simulink model "wqRL_multi_bal_system"  (R2021a)
settings: Solver=ode23t  StartTime=0.0  StopTime=Inf  FixedStep=0.02  RelTol=1e-3  AbsTol=1e-3
undefined symbols (not defined in the file or in its folder): dphi0, dtheta0, phi0, Tf, theta0, Ts
libraries: angle_lib x4, simulink_extras x2, pendulumLib x1, rllib x1, simulink x1
settings Model: DataDictionary=rl_data.sldd  Creator=tshintai  LastModifiedBy=WQ
settings SolverCC: AutoScaleAbsTol=off
settings ExplorerConfigSet: InternalSimMechanicsExplorerSettings="<ExplorerConfiguration><canonicalview>default</canonicalview><AnimationSetting><BasePlaybackSpeed>1.0</BasePlaybackSpeed><PlaybackSpeedFactor>1.0</PlaybackSpeedFactor></AnimationSetting><TilePanel><TileInfo><Tiles Columns=\"1\" Count=\"1\" Rows=\"1\"><Column Weight=\"1\"/><Row Weight=\"1\"/><Tile Height=\"1\" Width=\"1\" X=\"0\" Y=\"0\"/></Tiles></TileInfo><SceneInfo><SceneViewer><BGColor><R>0.60000002384185791</R><G>0.60000002384185791</G><B>0.60000002384185791</B></BGColor><Camera><DoPerspective>on</DoPerspective><Position><X>0.334156231583514596</X><Y>0.107146061295956732</Y><Z>0.154419804164132285</Z></Position><Center><X>0.145480827141795971</X><Y>0.0537418892551446009</Y><Z>0.077934111254939889</Z></Center><Up><X>-0.332530024195597795</X><Y>-0.157027945704575345</Y><Z>0.929927958110882913</Z></Up><ViewLimDist>1</ViewLimDist><YLim>0.466307658154998583</YLim><XLim>0.535390274177961367</XLim></Camera></SceneViewer></SceneInfo></TilePanel><MechEditorPanel><Cameras><Camera><Id>Camera1</Id><Value><Name>Camera1</Name><NativeCamera><PositionKeyframeSet/><CenterKeyframeSet/><UpVectorKeyframeSet/></NativeCamera></Value></Camera></Cameras><GfxPanelCameraMap><MapElement CameraMLId=\"Camera1\" GfxPanelIndex=\"0\"/></GfxPanelCameraMap><VideoCreator><PlaybackSpeedRatio>1.0</PlaybackSpeedRatio><FrameRate>30</FrameRate><VideoFormat>Motion JPEG AVI</VideoFormat><FrameSize>auto</FrameSize></VideoCreator></MechEditorPanel></ExplorerConfiguration>"

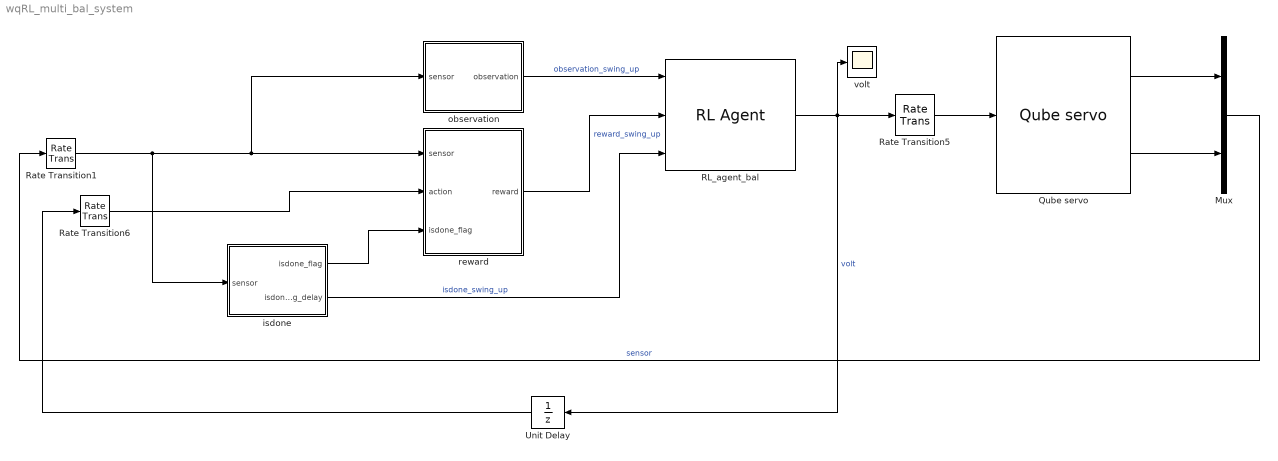
== system wqRL_multi_bal_system ==
  Mux : Mux  Inputs=2
  Qube servo : pendulumLib/Qube servo  a0=[theta0, phi0]  w0=[dtheta0, dphi0]  R_m=R_m  L_m=L_m  mu_m=mu_m  K_b=K_b_2  n=n  rod_mass=m_r  rod_length=L_r  rod_rad=rod_rad  p_mass=m_p  p_length=L_p  p_rad=p_rad  D_r=D_r_2  D_p=D_p
  RL_agent_bal : rllib/RL Agent  Agent=agent_bal  ExternalActionAsInput=off  ProvideCumRwd=off  TreatAsDirectFeedthrough=on
  Rate Transition1 : RateTransition  OutPortSampleTime=Ts
  Rate Transition5 : RateTransition
  Rate Transition6 : RateTransition  OutPortSampleTime=Ts
  Unit Delay : UnitDelay  SampleTime=-1  HasFrameUpgradeWarning=on
  isdone : Subsystem  VariantControl=VARIANT_INV_POS
  "observation " : Subsystem  VariantControl=VARIANT_OBS_ARM_PEND
  reward : Subsystem  VariantControl=VARIANT_INV_POS
  volt : Scope
  wires:
  Qube servo/1 -> Mux/1
  Qube servo/2 -> Mux/2
  Mux/1 -> Rate Transition1/1  "sensor"
  RL_agent_bal/1 -> Unit Delay/1, volt/1, Rate Transition5/1  "volt"
  Rate Transition5/1 -> Qube servo/1
  Unit Delay/1 -> Rate Transition6/1
  "observation "/1(observation) -> RL_agent_bal/1  "observation_swing_up"
  reward/1(reward) -> RL_agent_bal/2  "reward_swing_up"
  Rate Transition6/1 -> reward/2(action)
  isdone/2(isdone_flag_delay) -> RL_agent_bal/3  "isdone_swing_up"
  Rate Transition1/1 -> reward/1(sensor), "observation "/1(sensor), isdone/1(sensor)
  isdone/1(isdone_flag) -> reward/3(isdone_flag)

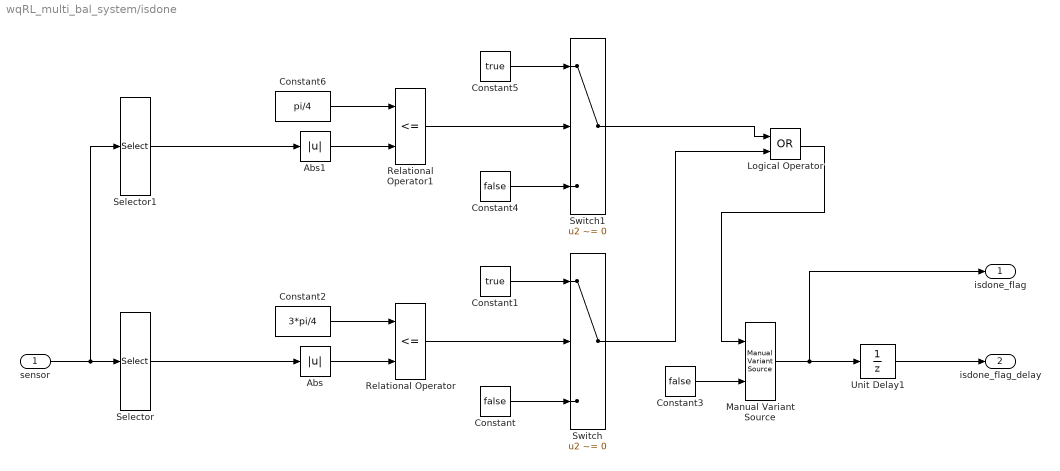
== system wqRL_multi_bal_system/isdone ==
  sensor : Inport
  Abs : Abs
  Abs1 : Abs
  Constant : Constant  Value=false
  Constant1 : Constant  Value=true
  Constant2 : Constant  Value=3*pi/4
  Constant3 : Constant  Value=false
  Constant4 : Constant  Value=false
  Constant5 : Constant  Value=true
  Constant6 : Constant  Value=pi/4
  Logical Operator : Logic  Operator=OR  AllPortsSameDT=off  OutDataTypeStr=boolean
  Manual Variant Source : simulink/Signal Routing/Manual Variant Source  NumChoices=2  LabelModeActiveChoice=V_2
  Relational Operator : RelationalOperator  Operator=<=  OutDataTypeStr=boolean  RndMeth=Simplest
  Relational Operator1 : RelationalOperator  Operator=<=  OutDataTypeStr=boolean  RndMeth=Simplest
  Selector : Selector  InputPortWidth=4  IndexOptions=Index vector (dialog)  Indices=[1]  OutputSizes=1
  Selector1 : Selector  InputPortWidth=4  IndexOptions=Index vector (dialog)  Indices=[2]  OutputSizes=1
  Switch : Switch  Criteria=u2 ~= 0
  Switch1 : Switch  Criteria=u2 ~= 0
  Unit Delay1 : UnitDelay  SampleTime=-1  HasFrameUpgradeWarning=on
  isdone_flag : Outport
  isdone_flag_delay : Outport  Port=2
  wires:
  Constant2/1 -> Relational Operator/1
  Constant/1 -> Switch/3
  Relational Operator/1 -> Switch/2
  Abs/1 -> Relational Operator/2
  Constant1/1 -> Switch/1
  Selector/1 -> Abs/1
  Switch/1 -> Logical Operator/2
  Manual Variant Source/1 -> isdone_flag/1, Unit Delay1/1
  Constant3/1 -> Manual Variant Source/2
  Unit Delay1/1 -> isdone_flag_delay/1
  Constant5/1 -> Switch1/1
  Switch1/1 -> Logical Operator/1
  Abs1/1 -> Relational Operator1/2
  Constant6/1 -> Relational Operator1/1
  Constant4/1 -> Switch1/3
  Relational Operator1/1 -> Switch1/2
  Selector1/1 -> Abs1/1
  sensor/1 -> Selector1/1, Selector/1
  Logical Operator/1 -> Manual Variant Source/1

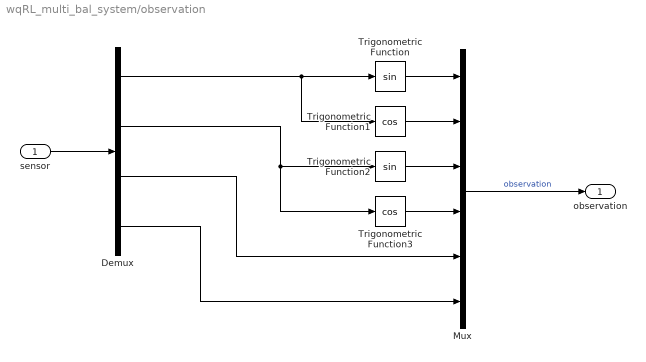
== system wqRL_multi_bal_system/observation  ==
  sensor : Inport
  Demux : Demux
  Mux : Mux  Inputs=6
  Trigonometric Function : Trigonometry
  Trigonometric Function1 : Trigonometry  Operator=cos
  Trigonometric Function2 : Trigonometry
  Trigonometric Function3 : Trigonometry  Operator=cos
  observation : Outport
  wires:
  Demux/4 -> Mux/6
  Demux/2 -> Trigonometric Function2/1, Trigonometric Function3/1
  Trigonometric Function3/1 -> Mux/4
  Trigonometric Function2/1 -> Mux/3
  sensor/1 -> Demux/1
  Mux/1 -> observation/1  "observation"
  Trigonometric Function/1 -> Mux/1
  Trigonometric Function1/1 -> Mux/2
  Demux/1 -> Trigonometric Function/1, Trigonometric Function1/1
  Demux/3 -> Mux/5

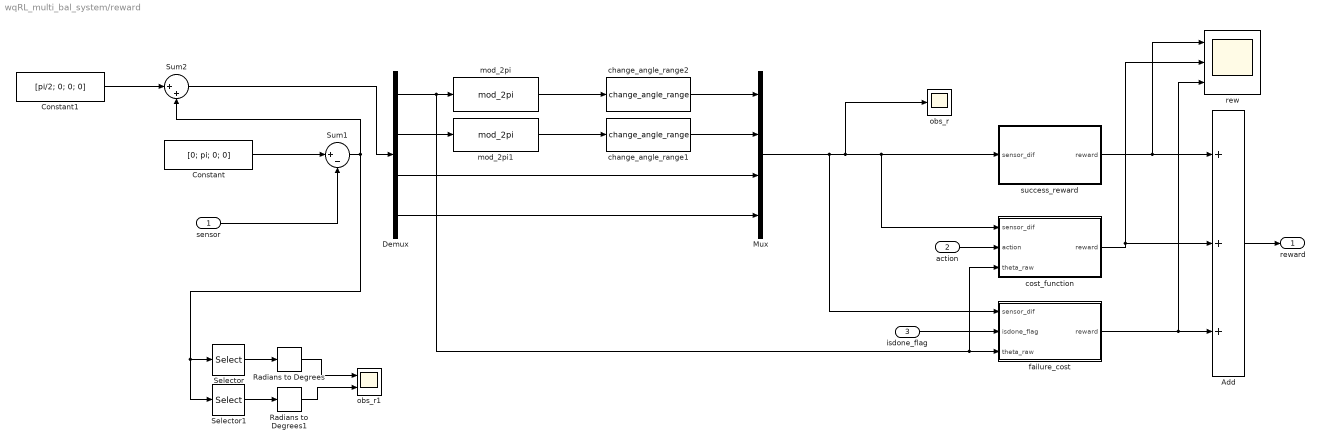
== system wqRL_multi_bal_system/reward ==
  sensor : Inport
  action : Inport  Port=2
  isdone_flag : Inport  Port=3
  Add : Sum  Inputs=+++
  Constant : Constant  Value=[0; pi; 0; 0]
  Constant1 : Constant  Value=[pi/2; 0; 0; 0]
  Demux : Demux
  Mux : Mux
  Radians to Degrees : simulink_extras/Transformations/Radians to Degrees
  Radians to Degrees1 : simulink_extras/Transformations/Radians to Degrees
  Selector : Selector  InputPortWidth=4  IndexOptions=Index vector (dialog)  Indices=[1]  OutputSizes=1
  Selector1 : Selector  InputPortWidth=4  IndexOptions=Index vector (dialog)  Indices=[2]  OutputSizes=1
  Sum1 : Sum  Inputs=|+-
  Sum2 : Sum  Inputs=|++
  change_angle_range1 : angle_lib/change_angle_range  SystemSampleTime=-1  VariantActivationTime=update diagram  Latency=0  AutoFrameSizeCalculation=off
  change_angle_range2 : angle_lib/change_angle_range  SystemSampleTime=-1  VariantActivationTime=update diagram  Latency=0  AutoFrameSizeCalculation=off
  cost_function : Subsystem
  failure_cost : Subsystem
  mod_2pi : angle_lib/mod_2pi  SystemSampleTime=-1  VariantActivationTime=update diagram  Latency=0  AutoFrameSizeCalculation=off
  mod_2pi1 : angle_lib/mod_2pi  SystemSampleTime=-1  VariantActivationTime=update diagram  Latency=0  AutoFrameSizeCalculation=off
  obs_r : Scope
  obs_r1 : Scope  NumInputPorts=2
  rew : Scope  NumInputPorts=3
  success_reward : Subsystem
  reward : Outport
  wires:
  isdone_flag/1 -> failure_cost/2(isdone_flag)
  failure_cost/1(reward) -> rew/3, Add/3
  success_reward/1(reward) -> rew/1, Add/1
  cost_function/1(reward) -> rew/2, Add/2
  action/1 -> cost_function/2(action)
  Add/1 -> reward/1
  Mux/1 -> cost_function/1(sensor_dif), success_reward/1(sensor_dif), obs_r/1, failure_cost/1(sensor_dif)
  Demux/2 -> mod_2pi1/1
  change_angle_range2/1 -> Mux/1
  change_angle_range1/1 -> Mux/2
  Demux/3 -> Mux/3
  Demux/4 -> Mux/4
  mod_2pi/1 -> change_angle_range2/1
  mod_2pi1/1 -> change_angle_range1/1
  Demux/1 -> failure_cost/3(theta_raw), cost_function/3(theta_raw), mod_2pi/1
  Radians to Degrees/1 -> obs_r1/1
  Radians to Degrees1/1 -> obs_r1/2
  Selector1/1 -> Radians to Degrees1/1
  Selector/1 -> Radians to Degrees/1
  sensor/1 -> Sum1/2
  Constant/1 -> Sum1/1
  Constant1/1 -> Sum2/1
  Sum1/1 -> Sum2/2, Selector1/1, Selector/1
  Sum2/1 -> Demux/1

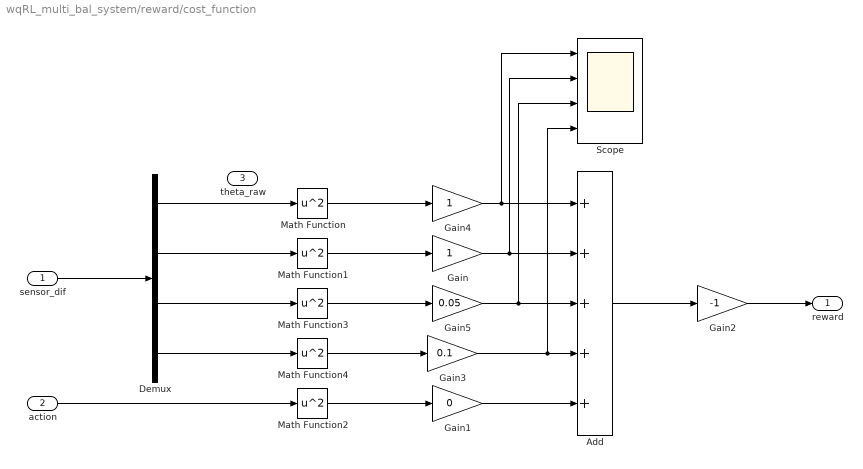
== system wqRL_multi_bal_system/reward/cost_function ==
  sensor_dif : Inport
  action : Inport  Port=2
  theta_raw : Inport  Port=3
  Add : Sum  Inputs=+++++
  Demux : Demux
  Gain : Gain
  Gain1 : Gain  Gain=0
  Gain2 : Gain  Gain=-1
  Gain3 : Gain  Gain=0.1
  Gain4 : Gain
  Gain5 : Gain  Gain=0.05
  Math Function{,1..4} (5 alike) : Math  Operator=square  SaturateOnIntegerOverflow=on
  Scope : Scope  NumInputPorts=4
  reward : Outport
  wires:
  Math Function4/1 -> Gain3/1
  Gain4/1 -> Scope/1, Add/1
  Gain/1 -> Scope/2, Add/2
  Gain5/1 -> Scope/3, Add/3
  Gain3/1 -> Scope/4, Add/4
  Gain1/1 -> Add/5
  Gain2/1 -> reward/1
  Add/1 -> Gain2/1
  sensor_dif/1 -> Demux/1
  Demux/4 -> Math Function4/1
  Demux/3 -> Math Function3/1
  Demux/2 -> Math Function1/1
  Math Function1/1 -> Gain/1
  Math Function3/1 -> Gain5/1
  action/1 -> Math Function2/1
  Demux/1 -> Math Function/1
  Math Function/1 -> Gain4/1
  Math Function2/1 -> Gain1/1

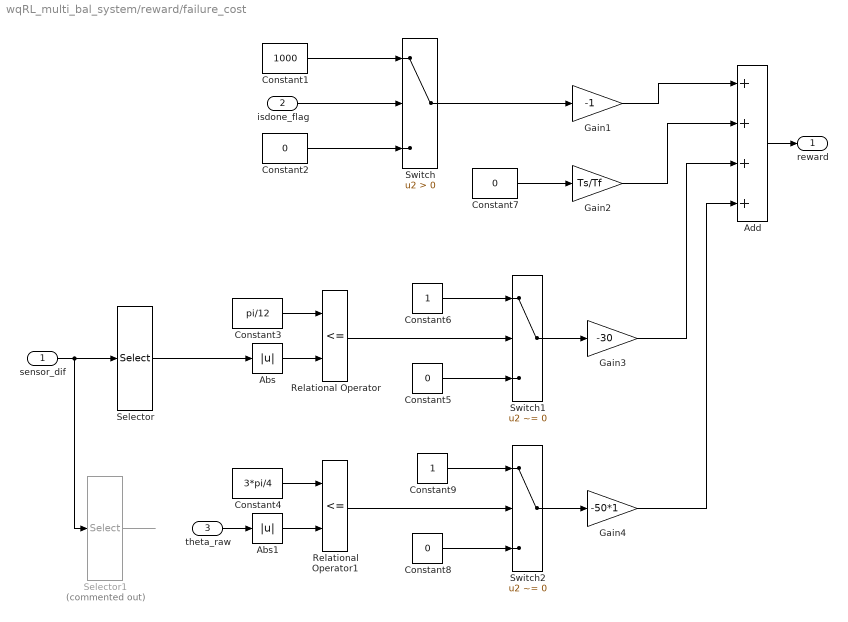
== system wqRL_multi_bal_system/reward/failure_cost ==
  sensor_dif : Inport
  isdone_flag : Inport  Port=2
  theta_raw : Inport  Port=3
  Abs : Abs
  Abs1 : Abs
  Add : Sum  Inputs=++++
  Constant1 : Constant  Value=1000
  Constant{2,5,7..8} (4 alike) : Constant  Value=0
  Constant3 : Constant  Value=pi/12
  Constant4 : Constant  Value=3*pi/4
  Constant6 : Constant
  Constant9 : Constant
  Gain1 : Gain  Gain=-1
  Gain2 : Gain  Gain=Ts/Tf
  Gain3 : Gain  Gain=-30
  Gain4 : Gain  Gain=-50*1
  Relational Operator : RelationalOperator  Operator=<=  OutDataTypeStr=boolean  RndMeth=Simplest
  Relational Operator1 : RelationalOperator  Operator=<=  OutDataTypeStr=boolean  RndMeth=Simplest
  Selector : Selector  InputPortWidth=4  IndexOptions=Index vector (dialog)  Indices=[2]  OutputSizes=1
  Selector1 : Selector  Commented=on  InputPortWidth=4  IndexOptions=Index vector (dialog)  Indices=[1]  OutputSizes=1
  Switch : Switch  Criteria=u2 > Threshold
  Switch1 : Switch  Criteria=u2 ~= 0
  Switch2 : Switch  Criteria=u2 ~= 0
  reward : Outport
  wires:
  Gain1/1 -> Add/1
  Constant2/1 -> Switch/3
  Constant1/1 -> Switch/1
  isdone_flag/1 -> Switch/2
  Switch/1 -> Gain1/1
  Gain2/1 -> Add/2
  Add/1 -> reward/1
  Constant7/1 -> Gain2/1
  Gain3/1 -> Add/3
  Abs/1 -> Relational Operator/2
  Constant5/1 -> Switch1/3
  Switch1/1 -> Gain3/1
  Relational Operator/1 -> Switch1/2
  Constant6/1 -> Switch1/1
  Selector/1 -> Abs/1
  Constant3/1 -> Relational Operator/1
  Gain4/1 -> Add/4
  Switch2/1 -> Gain4/1
  Constant8/1 -> Switch2/3
  Selector1/1 -> ?
  sensor_dif/1 -> Selector1/1, Selector/1
  Relational Operator1/1 -> Switch2/2
  theta_raw/1 -> Abs1/1
  Constant4/1 -> Relational Operator1/1
  Abs1/1 -> Relational Operator1/2
  Constant9/1 -> Switch2/1

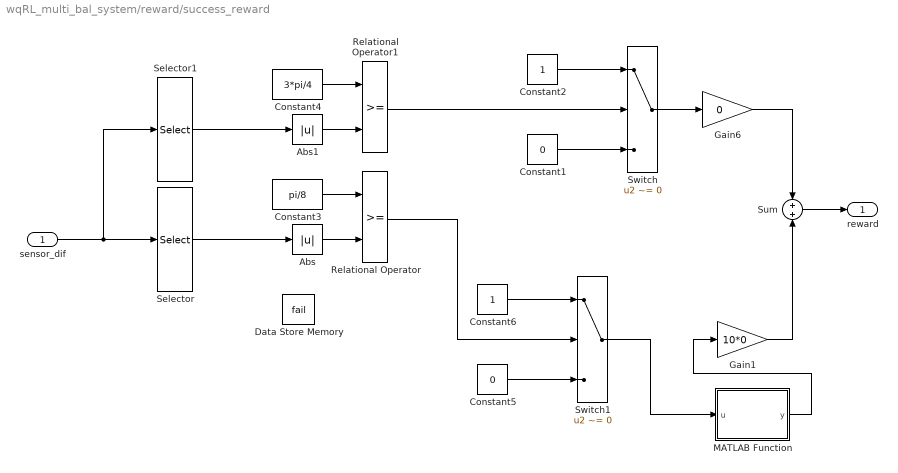
== system wqRL_multi_bal_system/reward/success_reward ==
  sensor_dif : Inport
  Abs : Abs
  Abs1 : Abs
  Constant1 : Constant  Value=0
  Constant2 : Constant
  Constant3 : Constant  Value=pi/8
  Constant4 : Constant  Value=3*pi/4
  Constant5 : Constant  Value=0
  Constant6 : Constant
  Data Store Memory : DataStoreMemory  DataStoreName=fail  ReadBeforeWriteMsg=warning  WriteAfterWriteMsg=warning  WriteAfterReadMsg=warning  ShowAdditionalParam=off  OutDataTypeStr=double
  Gain1 : Gain  Gain=10*0
  Gain6 : Gain  Gain=0
  MATLAB Function : MATLAB Function  TreatAsAtomicUnit=on
  Relational Operator : RelationalOperator  OutDataTypeStr=boolean  RndMeth=Simplest
  Relational Operator1 : RelationalOperator  OutDataTypeStr=boolean  RndMeth=Simplest
  Selector : Selector  InputPortWidth=4  IndexOptions=Index vector (dialog)  Indices=[2]  OutputSizes=1
  Selector1 : Selector  InputPortWidth=4  IndexOptions=Index vector (dialog)  Indices=[1]  OutputSizes=1
  Sum : Sum  Inputs=+|+
  Switch : Switch  Criteria=u2 ~= 0
  Switch1 : Switch  Criteria=u2 ~= 0
  reward : Outport
  wires:
  sensor_dif/1 -> Selector1/1, Selector/1
  Gain6/1 -> Sum/1
  Selector/1 -> Abs/1
  Constant2/1 -> Switch/1
  Constant1/1 -> Switch/3
  Switch/1 -> Gain6/1
  Constant3/1 -> Relational Operator/1
  Abs/1 -> Relational Operator/2
  Relational Operator1/1 -> Switch/2
  Abs1/1 -> Relational Operator1/2
  Constant4/1 -> Relational Operator1/1
  Selector1/1 -> Abs1/1
  Relational Operator/1 -> Switch1/2
  Switch1/1 -> MATLAB Function/1(u)
  Constant5/1 -> Switch1/3
  Constant6/1 -> Switch1/1
  Gain1/1 -> Sum/2
  Sum/1 -> reward/1
  MATLAB Function/1(y) -> Gain1/1

== matlab function wqRL_multi_bal_system/reward/success_reward/MATLAB Function ==
  data: u input; y output; fail data_store_memory
function y = fcn(u)
global fail;
if (u==0)
    fail=1;
end

if (fail==1)
    y=0;
else
    y=1;
end
